simulink model "ejemplo_dis"  (R2020b)
settings: Solver=VariableStepAuto  StartTime=0.0  StopTime=1.5  RelTol=1e-3
values from neighbouring files (symbols this model uses):
  Ts = 1/50    (= 0.02)    [ejemplo_1_dis.m]    (also in mapeo_s2z.m = 0.1)
  wn = 4/(Ts*e)    [ejemplo_1_dis.m]    (also in mapeo_s2z.m = 0:1:pi/Ts)
libraries: dspsigops x2
settings Model: Creator=Acer  LastModifiedBy=Acer

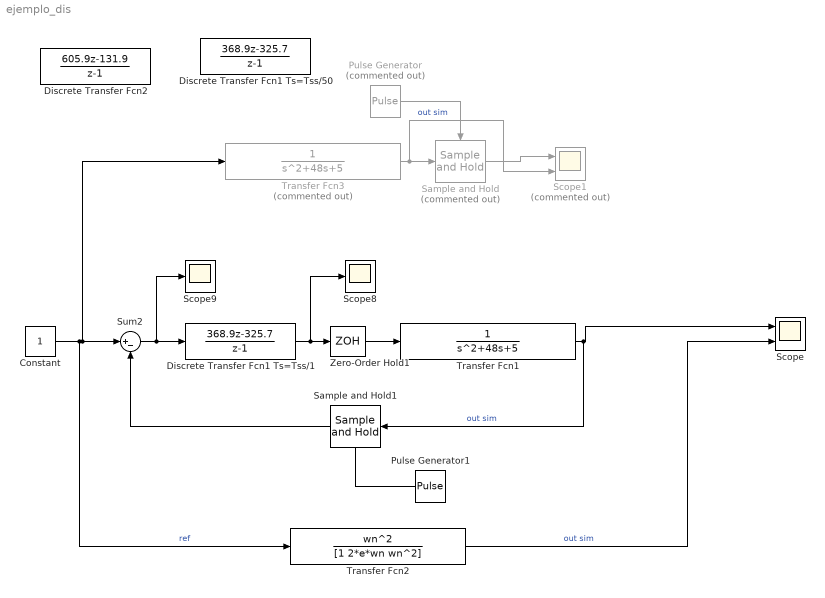
== system ejemplo_dis ==
  Constant : Constant
  Discrete Transfer Fcn1 Ts=Tss/1 : DiscreteTransferFcn  Numerator=[368.9 -325.7]  Denominator=[1 -1]  SampleTime=Ts
  Discrete Transfer Fcn1 Ts=Tss/50 : DiscreteTransferFcn  Numerator=[368.9 -325.7]  Denominator=[1 -1]  SampleTime=Ts
  Discrete Transfer Fcn2 : DiscreteTransferFcn  Numerator=[605.9 -131.9]  Denominator=[1 -1]  SampleTime=Ts
  Pulse Generator : DiscretePulseGenerator  Commented=on  PulseType=Time based  Period=Ts  PulseWidth=50
  Pulse Generator1 : DiscretePulseGenerator  PulseType=Time based  Period=Ts  PulseWidth=50
  Sample and Hold : dspsigops/Sample and Hold  Commented=on  trig=Rising edge  initCond=0  latchinput=off
  Sample and Hold1 : dspsigops/Sample and Hold  trig=Rising edge  initCond=0  latchinput=off
  Scope : Scope  NumInputPorts=2
  Scope1 : Scope  Commented=on  NumInputPorts=2
  Scope8 : Scope
  Scope9 : Scope
  Sum2 : Sum  Inputs=|+-
  Transfer Fcn1 : TransferFcn  Denominator=[1 48 5]
  Transfer Fcn2 : TransferFcn  Numerator=wn^2  Denominator=[1 2*e*wn wn^2]
  Transfer Fcn3 : TransferFcn  Commented=on  Denominator=[1 48 5]
  Zero-Order Hold1 : ZeroOrderHold  SampleTime=Ts
  wires:
  Discrete Transfer Fcn1 Ts=Tss/1/1 -> Zero-Order Hold1/1, Scope8/1
  Transfer Fcn1/1 -> Sample and Hold1/1, Scope/1  "out sim"
  Sum2/1 -> Discrete Transfer Fcn1 Ts=Tss/1/1, Scope9/1
  Constant/1 -> Transfer Fcn2/1, Transfer Fcn3/1, Sum2/1  "ref"
  Zero-Order Hold1/1 -> Transfer Fcn1/1
  Transfer Fcn2/1 -> Scope/2  "out sim"
  Pulse Generator/1 -> Sample and Hold/Trigger
  Transfer Fcn3/1 -> Scope1/2, Sample and Hold/1  "out sim"
  Sample and Hold/1 -> Scope1/1
  Pulse Generator1/1 -> Sample and Hold1/Trigger
  Sample and Hold1/1 -> Sum2/2
